simulink model "Lab8"  (R2025b)
settings: Solver=VariableStepAuto  StartTime=0.0  StopTime=100  RelTol=1e-3
settings Model: Creator=title  LastModifiedBy=Wingshingsho

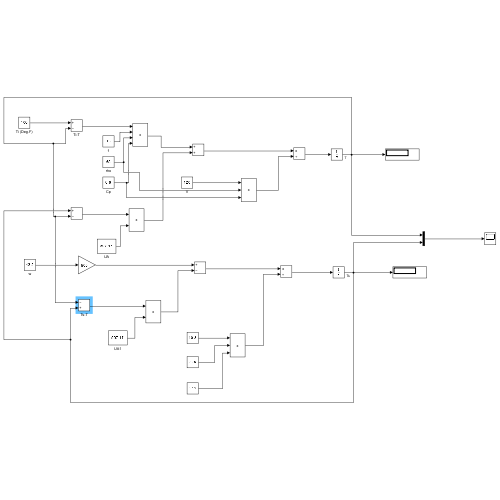
[thumbnail: Simulink's stored preview of the top-level diagram]
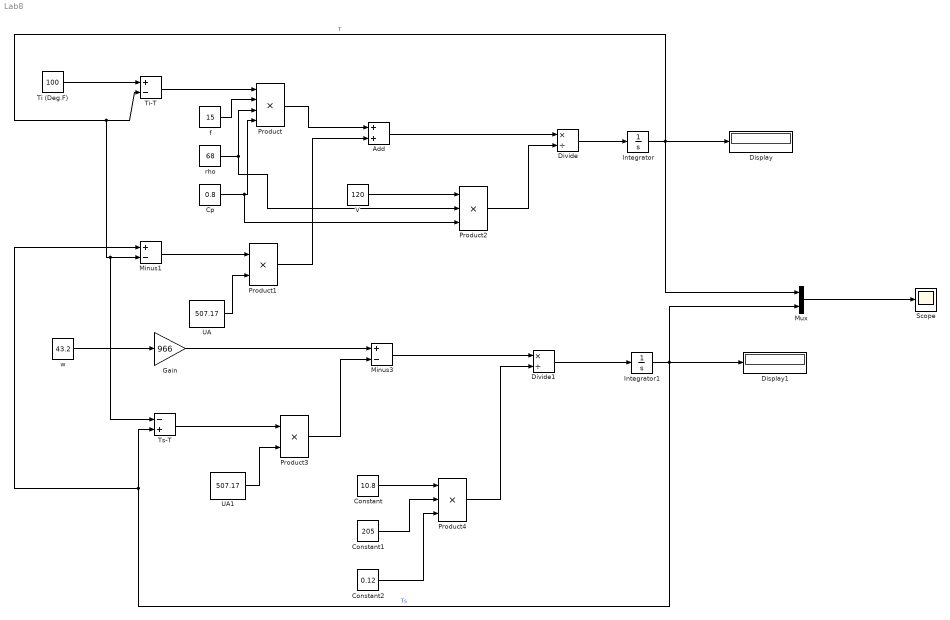
== system Lab8 ==
  Add : Sum
  Constant : Constant  Value=10.8
  Constant1 : Constant  Value=205
  Constant2 : Constant  Value=0.12
  Cp : Constant  Value=0.8
  Display : Display
  Display1 : Display
  Divide : Product  Inputs=*/
  Divide1 : Product  Inputs=*/
  Gain : Gain  Gain=966
  Integrator : Integrator
  Integrator1 : Integrator
  Minus1 : Sum  Inputs=+-
  Minus3 : Sum  Inputs=+-
  Mux : Mux  Inputs=2
  Product : Product  Inputs=4
  Product1 : Product
  Product2 : Product  Inputs=3
  Product3 : Product
  Product4 : Product  Inputs=3
  Scope : Scope
      settings: ActiveDisplayYMinimum=-29.174227213169566  ActiveDisplayYMaximum=262.56804491852614
  Ti (Deg.F) : Constant  Value=100
  Ti-T : Sum  Inputs=+-
  Ts-T : Sum  Inputs=-+
  UA : Constant  Value=507.17
  UA1 : Constant  Value=507.17
  V : Constant  Value=120
  f : Constant  Value=15
  rho : Constant  Value=68
  w : Constant  Value=43.2
  wires:
  Ti (Deg.F)/1 -> Ti-T/1
  Ti-T/1 -> Product/1
  f/1 -> Product/2
  rho/1 -> Product/3, Product2/2
  Minus1/1 -> Product1/1
  UA/1 -> Product1/2
  Product/1 -> Add/1
  Product1/1 -> Add/2
  Cp/1 -> Product2/3, Product/4
  V/1 -> Product2/1
  Add/1 -> Divide/1
  Product2/1 -> Divide/2
  Divide/1 -> Integrator/1
  Integrator/1 -> Mux/1, Display/1, Ti-T/2, Minus1/2, Ts-T/1  "T"
  w/1 -> Gain/1
  Ts-T/1 -> Product3/1
  UA1/1 -> Product3/2
  Gain/1 -> Minus3/1
  Product3/1 -> Minus3/2
  Constant/1 -> Product4/1
  Constant1/1 -> Product4/2
  Constant2/1 -> Product4/3
  Minus3/1 -> Divide1/1
  Product4/1 -> Divide1/2
  Divide1/1 -> Integrator1/1
  Integrator1/1 -> Mux/2, Display1/1, Ts-T/2, Minus1/1  "Ts"
  Mux/1 -> Scope/1
